simulink model "AudioFilterSystem"  (R2025a)
settings: Solver=VariableStepAuto  StartTime=0.0  StopTime=10.0  RelTol=1e-3
settings Model: DataDictionary=AudioFilterSystem_dict.sldd  Creator=morqu  LastModifiedBy=morqu

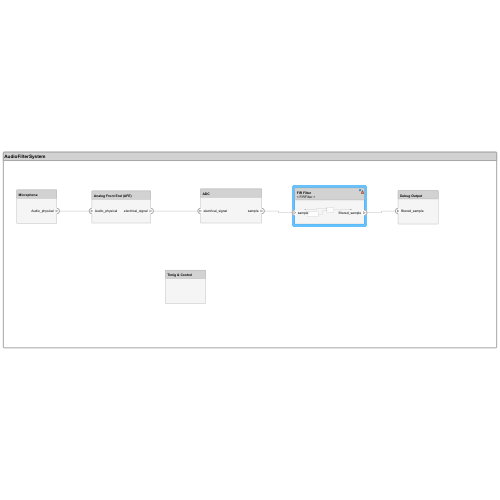
[thumbnail: Simulink's stored preview of the top-level diagram]
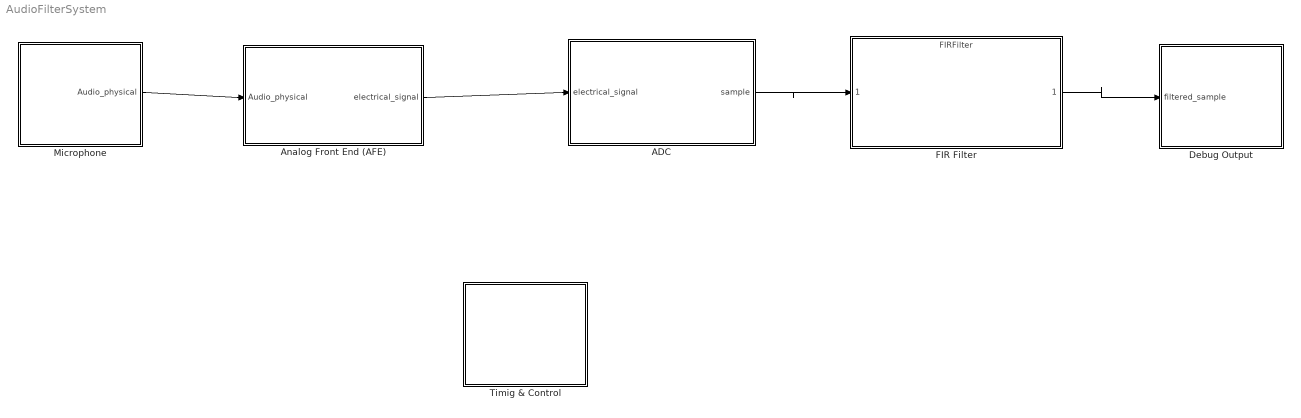
== system AudioFilterSystem ==
  ADC : Subsystem
      settings: PortSchema="{\"entries\":[{\"content\":{\"headerSize\":26,\"margin\":15,\"minimumSpacing\":25,\"sides\":[{\"content\":{\"connectorIds\":[\"In1\"]},\"type\":\"ConnectorPlacement.EquallySpacedRectSide\",\"uuid\":\"994861de-6d69-4d68-a178-d0521cde0fd8\"},{\"content\":{\"connectorIds\":[\"Out1\"],\"side\":\"RIGHT\"},\"type\":\"ConnectorPlacement.EquallySpacedRectSide\",\"uuid\":\"1da4d04f-7762-4bd1-96dc-038b62a5db96\"},{\"content\":{\"side\":\"TOP\"},\"type\":\"ConnectorPlacement.EquallySpacedRectSide\",\"uuid\":\"22be2d7f-4c17-4466-9c74-63d2aa215182\"}]},\"type\":\"ConnectorPlacement.EquallySpacedConnector\",\"uuid\":\"a1c2c75d-8205-41be-97fd-48d1178e575e\"}],\"packageUris\":[\"http://schema.mathworks.com/mf0/Connector/R2020b\"],\"version\":\"1.0\"}"
  Analog Front End (AFE) : Subsystem
      settings: PortSchema="{\"entries\":[{\"content\":{\"headerSize\":26,\"margin\":15,\"minimumSpacing\":25,\"sides\":[{\"content\":{\"connectorIds\":[\"In1\"]},\"type\":\"ConnectorPlacement.EquallySpacedRectSide\",\"uuid\":\"994861de-6d69-4d68-a178-d0521cde0fd8\"},{\"content\":{\"connectorIds\":[\"Out1\"],\"side\":\"RIGHT\"},\"type\":\"ConnectorPlacement.EquallySpacedRectSide\",\"uuid\":\"1da4d04f-7762-4bd1-96dc-038b62a5db96\"},{\"content\":{\"side\":\"TOP\"},\"type\":\"ConnectorPlacement.EquallySpacedRectSide\",\"uuid\":\"22be2d7f-4c17-4466-9c74-63d2aa215182\"}]},\"type\":\"ConnectorPlacement.EquallySpacedConnector\",\"uuid\":\"a1c2c75d-8205-41be-97fd-48d1178e575e\"}],\"packageUris\":[\"http://schema.mathworks.com/mf0/Connector/R2020b\"],\"version\":\"1.0\"}"
  Debug Output : Subsystem
      settings: PortSchema="{\"entries\":[{\"content\":{\"headerSize\":26,\"margin\":15,\"minimumSpacing\":25,\"sides\":[{\"content\":{\"connectorIds\":[\"In1\"]},\"type\":\"ConnectorPlacement.EquallySpacedRectSide\",\"uuid\":\"994861de-6d69-4d68-a178-d0521cde0fd8\"},{\"content\":{\"side\":\"RIGHT\"},\"type\":\"ConnectorPlacement.EquallySpacedRectSide\",\"uuid\":\"1da4d04f-7762-4bd1-96dc-038b62a5db96\"},{\"content\":{\"side\":\"TOP\"},\"type\":\"ConnectorPlacement.EquallySpacedRectSide\",\"uuid\":\"22be2d7f-4c17-4466-9c74-63d2aa215182\"}]},\"type\":\"ConnectorPlacement.EquallySpacedConnector\",\"uuid\":\"a1c2c75d-8205-41be-97fd-48d1178e575e\"}],\"packageUris\":[\"http://schema.mathworks.com/mf0/Connector/R2020b\"],\"version\":\"1.0\"}"
  FIR Filter : ModelReference  ModelNameDialog=FIRFilter  SimulationMode=Normal  ModelReferenceVersion=1.2
      settings: PortSchema="{\"entries\":[{\"content\":{\"headerSize\":38,\"margin\":15,\"minimumSpacing\":25,\"sides\":[{\"content\":{\"connectorIds\":[\"In1\"]},\"type\":\"ConnectorPlacement.EquallySpacedRectSide\",\"uuid\":\"994861de-6d69-4d68-a178-d0521cde0fd8\"},{\"content\":{\"connectorIds\":[\"Out1\"],\"side\":\"RIGHT\"},\"type\":\"ConnectorPlacement.EquallySpacedRectSide\",\"uuid\":\"1da4d04f-7762-4bd1-96dc-038b62a5db96\"},{\"content\":{\"side\":\"TOP\"},\"type\":\"ConnectorPlacement.EquallySpacedRectSide\",\"uuid\":\"22be2d7f-4c17-4466-9c74-63d2aa215182\"}]},\"type\":\"ConnectorPlacement.EquallySpacedConnector\",\"uuid\":\"a1c2c75d-8205-41be-97fd-48d1178e575e\"}],\"packageUris\":[\"http://schema.mathworks.com/mf0/Connector/R2020b\"],\"version\":\"1.0\"}"
  Microphone : Subsystem
      settings: PortSchema="{\"entries\":[{\"content\":{\"headerSize\":26,\"margin\":15,\"minimumSpacing\":25,\"sides\":[{\"content\":{},\"type\":\"ConnectorPlacement.EquallySpacedRectSide\",\"uuid\":\"994861de-6d69-4d68-a178-d0521cde0fd8\"},{\"content\":{\"connectorIds\":[\"Out1\"],\"side\":\"RIGHT\"},\"type\":\"ConnectorPlacement.EquallySpacedRectSide\",\"uuid\":\"1da4d04f-7762-4bd1-96dc-038b62a5db96\"},{\"content\":{\"side\":\"TOP\"},\"type\":\"ConnectorPlacement.EquallySpacedRectSide\",\"uuid\":\"22be2d7f-4c17-4466-9c74-63d2aa215182\"}]},\"type\":\"ConnectorPlacement.EquallySpacedConnector\",\"uuid\":\"a1c2c75d-8205-41be-97fd-48d1178e575e\"}],\"packageUris\":[\"http://schema.mathworks.com/mf0/Connector/R2020b\"],\"version\":\"1.0\"}"
  Timig & Control : Subsystem
      settings: PortSchema="{\"entries\":[{\"content\":{\"headerSize\":26,\"margin\":15,\"minimumSpacing\":25,\"sides\":[{\"content\":{},\"type\":\"ConnectorPlacement.EquallySpacedRectSide\",\"uuid\":\"994861de-6d69-4d68-a178-d0521cde0fd8\"},{\"content\":{\"side\":\"RIGHT\"},\"type\":\"ConnectorPlacement.EquallySpacedRectSide\",\"uuid\":\"1da4d04f-7762-4bd1-96dc-038b62a5db96\"},{\"content\":{\"side\":\"TOP\"},\"type\":\"ConnectorPlacement.EquallySpacedRectSide\",\"uuid\":\"22be2d7f-4c17-4466-9c74-63d2aa215182\"}]},\"type\":\"ConnectorPlacement.EquallySpacedConnector\",\"uuid\":\"a1c2c75d-8205-41be-97fd-48d1178e575e\"}],\"packageUris\":[\"http://schema.mathworks.com/mf0/Connector/R2020b\"],\"version\":\"1.0\"}"
  wires:
  Microphone/1(Audio_physical) -> Analog Front End (AFE)/1(Audio_physical)
  Analog Front End (AFE)/1(electrical_signal) -> ADC/1(electrical_signal)
  ADC/1(sample) -> FIR Filter/1
  FIR Filter/1 -> Debug Output/1(filtered_sample)

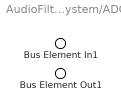
== system AudioFilterSystem/ADC ==
  Bus Element In1 : Inport  PortName=electrical_signal
  Bus Element Out1 : Outport  PortName=sample

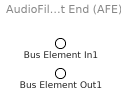
== system AudioFilterSystem/Analog Front End (AFE) ==
  Bus Element In1 : Inport  PortName=Audio_physical
  Bus Element Out1 : Outport  PortName=electrical_signal

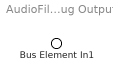
== system AudioFilterSystem/Debug Output ==
  Bus Element In1 : Inport  PortName=filtered_sample

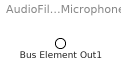
== system AudioFilterSystem/Microphone ==
  Bus Element Out1 : Outport  PortName=Audio_physical

== system AudioFilterSystem/Timig & Control ==
